simulink model "sf_superstep_cycle_error"  (Simulink 7.6)
settings: Solver=FixedStepDiscrete  StartTime=0.0  StopTime=10.0  FixedStep=1  RelTol=1e-3
settings Model: Creator=The MathWorks Inc.
settings OptimizationCC: InitFltsAndDblsToZero=on  EfficientMapNaN2IntZero=off
settings DebuggingCC: StrictBusMsg=Warning
settings SFSimCC: SimParseCustomCode=off

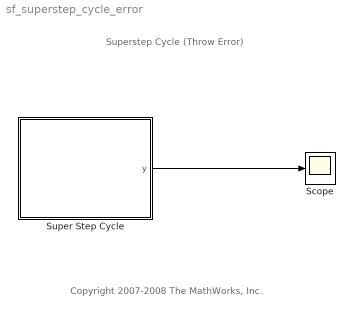
== system sf_superstep_cycle_error ==
  note: Superstep Cycle (Throw Error)
  note: Copyright 2007-2008 The MathWorks, Inc.
  Scope : Scope
  Super Step Cycle : Stateflow chart  TreatAsAtomicUnit=on
  wires:
  Super Step Cycle/1(y) -> Scope/1

== stateflow chart Super Step Cycle ==
  settings: enableNonTerminalStates=1
  state A
    en: y = 1;
  state B
    en: y = 2;
  A -> B : [ x == 1 ]
  B -> A
  (default) -> A : { x = 1; }
  data: y output double; x local double
